simulink model "biadler_sim_3_TEST"  (R2013a)
settings: Solver=ode1  StartTime=0.0  StopTime=5.11  FixedStep=0.001  MaxStep=0.01  RelTol=1e-3
libraries: simulink x4
settings Model: Creator=Administrator  LastModifiedBy=dholley
settings SolverCC: ExtrapolationOrder=1
settings DataIOCC: LimitDataPoints=off  SaveFormat=StructureWithTime  SignalLoggingSaveFormat=ModelDataLogs  SaveOutput=off  SignalLogging=off  DSMLogging=off  SaveTime=off
settings OptimizationCC: InlineParams=on  InlineInvariantSignals=on  ExpressionDepthLimit=2147483647  EfficientFloat2IntCast=on  SimCompilerOptimization=On
settings DebuggingCC: FcnCallInpInsideContextMsg=UseLocalSettings
settings HardwareCC: ProdIntDivRoundTo=Zero  ProdEndianess=LittleEndian  ProdHWDeviceType=Generic->32-bit x86 compatible  TargetIntDivRoundTo=Zero  TargetEndianess=LittleEndian  TargetHWDeviceType=MATLAB Host
settings ModelReferenceCC: ModelReferenceNumInstancesAllowed=Zero
settings RTWCC: SystemTargetFile=grt_malloc.tlc  TemplateMakefile=grt_malloc_default_tmf  Description=Generic Real-Time Target with dynamic memory allocation  RTWVerbose=off  ProcessScript=grt_malloc_make_rtw_hook  RTWCompilerOptimization=On
settings CodeAppCC: GenerateComments=off  SimulinkBlockComments=off
settings GRTTargetCC: CodeReplacementLibrary=C89/C90 (ANSI)  CombineOutputUpdateFcns=off  MatFileLogging=off  GRTInterface=on  UseMalloc=on  ExtModeMexFile=noextcomm

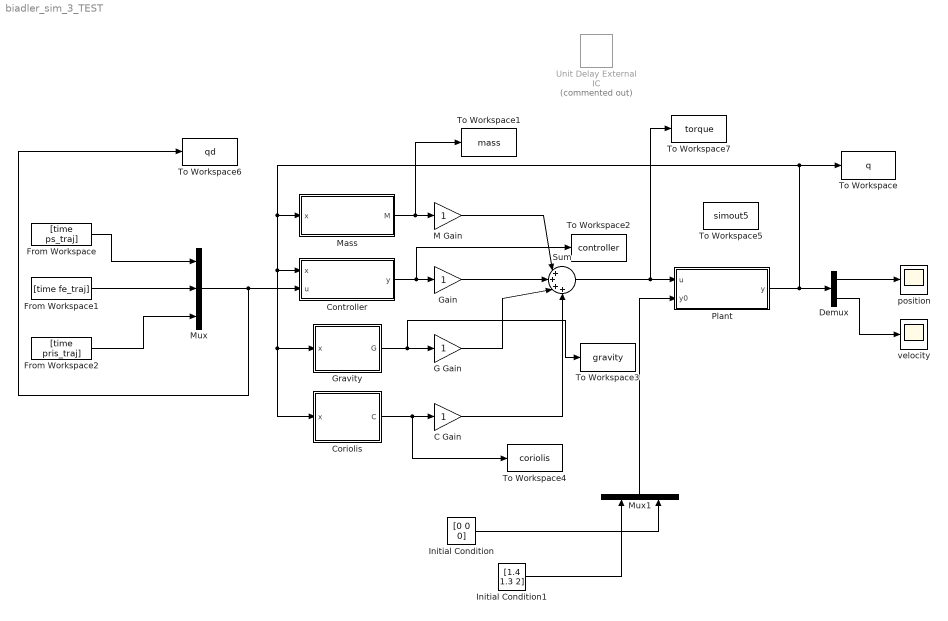
== system biadler_sim_3_TEST ==
  C Gain : Gain
  Controller : Subsystem  TreatAsAtomicUnit=on
  Coriolis : MATLAB Function  TreatAsAtomicUnit=on
  Demux : Demux  Outputs=2
  From Workspace : FromWorkspace  VariableName=[time ps_traj]  SampleTime=0
  From Workspace1 : FromWorkspace  VariableName=[time fe_traj]  SampleTime=0
  From Workspace2 : FromWorkspace  VariableName=[time pris_traj]  SampleTime=0
  G Gain : Gain
  Gain : Gain
  Gravity : MATLAB Function  TreatAsAtomicUnit=on
  Initial Condition : Constant  Value=[0 0 0]
  Initial Condition1 : Constant  Value=[1.4 1.3 2]
  M Gain : Gain
  Mass : Subsystem  TreatAsAtomicUnit=on
  Mux : Mux  Inputs=3
  Mux1 : Mux  Inputs=2
  Plant : Subsystem  TreatAsAtomicUnit=on
  Sum : Sum  Inputs=|++++
  To Workspace : ToWorkspace  VariableName=q  SampleTime=-1  SaveFormat=Timeseries
  To Workspace1 : ToWorkspace  VariableName=mass  SampleTime=-1  SaveFormat=Timeseries
  To Workspace2 : ToWorkspace  VariableName=controller  SampleTime=-1  SaveFormat=Timeseries
  To Workspace3 : ToWorkspace  VariableName=gravity  SampleTime=-1  SaveFormat=Timeseries
  To Workspace4 : ToWorkspace  VariableName=coriolis  SampleTime=-1  SaveFormat=Timeseries
  To Workspace5 : ToWorkspace  VariableName=simout5  SampleTime=-1  SaveFormat=Timeseries
  To Workspace6 : ToWorkspace  VariableName=qd  SampleTime=-1  SaveFormat=Timeseries
  To Workspace7 : ToWorkspace  VariableName=torque  SampleTime=-1  SaveFormat=Timeseries
  Unit Delay External IC : simulink/Additional Math & Discrete/Additional Discrete/Unit Delay External IC  Commented=on  tsamp=-1
  position : Scope
      settings: TickLabels=on  TimeRange=2  YMin=-3  YMax=3  SampleTime=0.05
  velocity : Scope
      settings: TickLabels=on  TimeRange=2  YMin=-1  YMax=1  SampleTime=0.05
  wires:
  Demux/2 -> velocity/1
  Plant/1(y) -> Demux/1, To Workspace/1, Mass/1(x), Controller/1(x), Gravity/1(x), Coriolis/1(x)
  Sum/1 -> To Workspace7/1, Plant/1(u)
  Gravity/1(G) -> To Workspace3/1, G Gain/1
  Coriolis/1(C) -> To Workspace4/1, C Gain/1
  C Gain/1 -> Sum/4
  M Gain/1 -> Sum/1
  G Gain/1 -> Sum/3
  Controller/1(y) -> To Workspace2/1, Gain/1
  Mass/1(M) -> To Workspace1/1, M Gain/1
  Gain/1 -> Sum/2
  Demux/1 -> position/1
  From Workspace/1 -> Mux/1
  From Workspace1/1 -> Mux/2
  From Workspace2/1 -> Mux/3
  Mux/1 -> To Workspace6/1, Controller/2(u)
  Initial Condition/1 -> Mux1/2
  Initial Condition1/1 -> Mux1/1
  Mux1/1 -> Plant/2(y0)

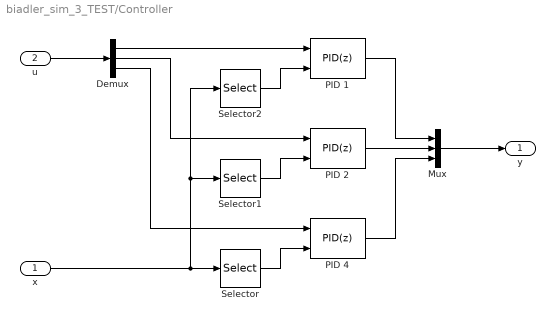
== system biadler_sim_3_TEST/Controller ==
  x : Inport
  u : Inport  Port=2
  Demux : Demux  Outputs=3
  Mux : Mux  Inputs=3
  PID 1 : simulink/Continuous/PID Controller (2DOF)  Controller=PID  TimeDomain=Discrete-time  SampleTime=0.001  IntegratorMethod=Forward Euler  FilterMethod=Forward Euler  Form=Parallel  P=2490  I=3860  D=163  N=250  b=1  c=1  InitialConditionSource=internal  InitialConditionForIntegrator=0  InitialConditionForFilter=0  ExternalReset=none  LimitOutput=off  UpperSaturationLimit=5  LowerSaturationLimit=-5  LinearizeAsGain=off  AntiWindupMode=none  Kb=1  TrackingMode=off  Kt=1  PParamMin=[]  PParamMax=[]  IParamMin=[]  IParamMax=[]  DParamMin=[]  DParamMax=[]  NParamMin=[]  NParamMax=[]  bParamMin=[]  bParamMax=[]  cParamMin=[]  cParamMax=[]  KbParamMin=[]  KbParamMax=[]  KtParamMin=[]  KtParamMax=[]  POutMin=[]  POutMax=[]  IOutMin=[]  IOutMax=[]  DOutMin=[]  DOutMax=[]  NOutMin=[]  NOutMax=[]  bOutMin=[]  bOutMax=[]  cOutMin=[]  cOutMax=[]  KbOutMin=[]  KbOutMax=[]  KtOutMin=[]  KtOutMax=[]  IntegratorOutMin=[]  IntegratorOutMax=[]  FilterOutMin=[]  FilterOutMax=[]  SumOutMin=[]  SumOutMax=[]  Sum1OutMin=[]  Sum1OutMax=[]  Sum2OutMin=[]  Sum2OutMax=[]  Sum3OutMin=[]  Sum3OutMax=[]  SumI1OutMin=[]  SumI1OutMax=[]  SumI2OutMin=[]  SumI2OutMax=[]  SumI3OutMin=[]  SumI3OutMax=[]  SumDOutMin=[]  SumDOutMax=[]  SaturationOutMin=[]  SaturationOutMax=[]  IntegratorContinuousStateAttributes=''  IntegratorStateMustResolveToSignalObject=off  IntegratorRTWStateStorageClass=Auto  FilterContinuousStateAttributes=''  FilterStateMustResolveToSignalObject=off  FilterRTWStateStorageClass=Auto
  PID 2 : simulink/Continuous/PID Controller (2DOF)  Controller=PID  TimeDomain=Discrete-time  SampleTime=0.001  IntegratorMethod=Forward Euler  FilterMethod=Forward Euler  Form=Parallel  P=2490  I=3860  D=163  N=250  b=1  c=1  InitialConditionSource=internal  InitialConditionForIntegrator=0  InitialConditionForFilter=0  ExternalReset=none  LimitOutput=off  UpperSaturationLimit=5  LowerSaturationLimit=-5  LinearizeAsGain=off  AntiWindupMode=none  Kb=1  TrackingMode=off  Kt=1  PParamMin=[]  PParamMax=[]  IParamMin=[]  IParamMax=[]  DParamMin=[]  DParamMax=[]  NParamMin=[]  NParamMax=[]  bParamMin=[]  bParamMax=[]  cParamMin=[]  cParamMax=[]  KbParamMin=[]  KbParamMax=[]  KtParamMin=[]  KtParamMax=[]  POutMin=[]  POutMax=[]  IOutMin=[]  IOutMax=[]  DOutMin=[]  DOutMax=[]  NOutMin=[]  NOutMax=[]  bOutMin=[]  bOutMax=[]  cOutMin=[]  cOutMax=[]  KbOutMin=[]  KbOutMax=[]  KtOutMin=[]  KtOutMax=[]  IntegratorOutMin=[]  IntegratorOutMax=[]  FilterOutMin=[]  FilterOutMax=[]  SumOutMin=[]  SumOutMax=[]  Sum1OutMin=[]  Sum1OutMax=[]  Sum2OutMin=[]  Sum2OutMax=[]  Sum3OutMin=[]  Sum3OutMax=[]  SumI1OutMin=[]  SumI1OutMax=[]  SumI2OutMin=[]  SumI2OutMax=[]  SumI3OutMin=[]  SumI3OutMax=[]  SumDOutMin=[]  SumDOutMax=[]  SaturationOutMin=[]  SaturationOutMax=[]  IntegratorContinuousStateAttributes=''  IntegratorStateMustResolveToSignalObject=off  IntegratorRTWStateStorageClass=Auto  FilterContinuousStateAttributes=''  FilterStateMustResolveToSignalObject=off  FilterRTWStateStorageClass=Auto
  PID 4 : simulink/Continuous/PID Controller (2DOF)  Controller=PID  TimeDomain=Discrete-time  SampleTime=0.001  IntegratorMethod=Forward Euler  FilterMethod=Forward Euler  Form=Parallel  P=2490  I=3860  D=163  N=250  b=1  c=1  InitialConditionSource=internal  InitialConditionForIntegrator=0  InitialConditionForFilter=0  ExternalReset=none  LimitOutput=off  UpperSaturationLimit=5  LowerSaturationLimit=-5  LinearizeAsGain=off  AntiWindupMode=none  Kb=1  TrackingMode=off  Kt=1  PParamMin=[]  PParamMax=[]  IParamMin=[]  IParamMax=[]  DParamMin=[]  DParamMax=[]  NParamMin=[]  NParamMax=[]  bParamMin=[]  bParamMax=[]  cParamMin=[]  cParamMax=[]  KbParamMin=[]  KbParamMax=[]  KtParamMin=[]  KtParamMax=[]  POutMin=[]  POutMax=[]  IOutMin=[]  IOutMax=[]  DOutMin=[]  DOutMax=[]  NOutMin=[]  NOutMax=[]  bOutMin=[]  bOutMax=[]  cOutMin=[]  cOutMax=[]  KbOutMin=[]  KbOutMax=[]  KtOutMin=[]  KtOutMax=[]  IntegratorOutMin=[]  IntegratorOutMax=[]  FilterOutMin=[]  FilterOutMax=[]  SumOutMin=[]  SumOutMax=[]  Sum1OutMin=[]  Sum1OutMax=[]  Sum2OutMin=[]  Sum2OutMax=[]  Sum3OutMin=[]  Sum3OutMax=[]  SumI1OutMin=[]  SumI1OutMax=[]  SumI2OutMin=[]  SumI2OutMax=[]  SumI3OutMin=[]  SumI3OutMax=[]  SumDOutMin=[]  SumDOutMax=[]  SaturationOutMin=[]  SaturationOutMax=[]  IntegratorContinuousStateAttributes=''  IntegratorStateMustResolveToSignalObject=off  IntegratorRTWStateStorageClass=Auto  FilterContinuousStateAttributes=''  FilterStateMustResolveToSignalObject=off  FilterRTWStateStorageClass=Auto
  Selector : Selector  InputPortWidth=6  IndexOptions=Index vector (dialog)  Indices=[3]  OutputSizes=1
  Selector1 : Selector  InputPortWidth=6  IndexOptions=Index vector (dialog)  Indices=[2]  OutputSizes=1
  Selector2 : Selector  InputPortWidth=6  IndexOptions=Index vector (dialog)  Indices=[1]  OutputSizes=1
  y : Outport
  wires:
  Selector2/1 -> PID 1/2
  Selector1/1 -> PID 2/2
  PID 2/1 -> Mux/2
  Mux/1 -> y/1
  PID 1/1 -> Mux/1
  PID 4/1 -> Mux/3
  x/1 -> Selector/1, Selector1/1, Selector2/1
  Demux/3 -> PID 4/1
  Demux/2 -> PID 2/1
  Demux/1 -> PID 1/1
  u/1 -> Demux/1
  Selector/1 -> PID 4/2

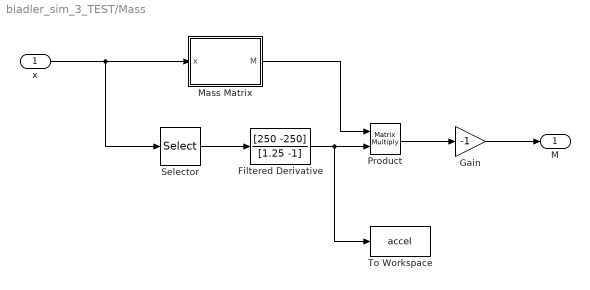
== system biadler_sim_3_TEST/Mass ==
  x : Inport
  Filtered Derivative : DiscreteFilter  Numerator=[250 -250]  Denominator=[1.25 -1]  SampleTime=0.001
  Gain : Gain  Gain=-1
  Mass Matrix : MATLAB Function  TreatAsAtomicUnit=on
  Product : Product  Multiplication=Matrix(*)  RndMeth=Zero
  Selector : Selector  InputPortWidth=6  IndexOptions=Index vector (dialog)  Indices=[4:6]  OutputSizes=1
  To Workspace : ToWorkspace  VariableName=accel  SampleTime=-1  SaveFormat=Timeseries
  M : Outport
  wires:
  x/1 -> Mass Matrix/1(x), Selector/1
  Filtered Derivative/1 -> To Workspace/1, Product/2
  Selector/1 -> Filtered Derivative/1
  Mass Matrix/1(M) -> Product/1
  Product/1 -> Gain/1
  Gain/1 -> M/1

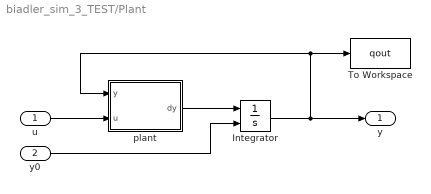
== system biadler_sim_3_TEST/Plant ==
  u : Inport
  y0 : Inport  Port=2
  Integrator : Integrator  InitialConditionSource=external  InitialCondition=[0;0;0.5;0;0;0]
  To Workspace : ToWorkspace  VariableName=qout  SampleTime=-1  SaveFormat=Structure With Time
  plant : MATLAB Function  TreatAsAtomicUnit=on
  y : Outport
  wires:
  Integrator/1 -> y/1, plant/1(y), To Workspace/1
  plant/1(dy) -> Integrator/1
  u/1 -> plant/2(u)
  y0/1 -> Integrator/2

== matlab function biadler_sim_3_TEST/Mass/Mass Matrix ==
  data: x input; M output
function M = fcn(x) %#codegen

I1=[0.38096322, 0.00007420, -0.00044613; 0.00007420, 0.33264110, -0.07673074; -0.00044613, -0.07673074, 0.05442464];
I2=[0.20019857, 0.11214860, -0.00179420; 0.11214860, 0.40696889, -0.00005073; -0.0017942, -0.00005073, 0.57750696];
I3=[0.25101842, -0.00000898, 0.00296055; -0.00000898, 0.24154846, 0.00011129; 0.00296055, 0.00011129, 0.01521556];
I23=I2+I3;

% m2=8.79496939;
m3=3.5;
% rg2=-0.12046546;
% rg3=-0.00429190;
% g=9.80665;

s2=sin(x(2)); c2=cos(x(2));

M=[(I1(3,3)+I23(1,1)*s2^2+I23(2,2)*c2^2-2*I23(1,2)*s2*c2+m3*x(3)*s2), (I23(1,3)*s2-I23(2,3)*c2), 0;
   (I23(1,3)*s2-I23(2,3)*c2), (I23(3,3)+m3*x(3)^2), 0;
   0, 0, m3];

== matlab function biadler_sim_3_TEST/Plant/plant ==
  data: y input; u input; dy output
function dy = fcn(y,u) %#codegen

I1=[0.38096322, 0.00007420, -0.00044613; 0.00007420, 0.33264110, -0.07673074; -0.00044613, -0.07673074, 0.05442464];
I2=[0.20019857, 0.11214860, -0.00179420; 0.11214860, 0.40696889, -0.00005073; -0.0017942, -0.00005073, 0.57750696];
I3=[0.25101842, -0.00000898, 0.00296055; -0.00000898, 0.24154846, 0.00011129; 0.00296055, 0.00011129, 0.01521556];
I23=I2+I3;

m2=8.79496939;
m3=3.5;
rg2=-0.12046546;
rg3=-0.00429190;
g=9.80665;

s2=sin(y(2)); c2=cos(y(2));

dyy=[y(4:6).^2;y(4)*y(5);y(5)*y(6);y(6)*y(4)];
C0=[0, (I23(1,3)*c2+I23(2,3)*s2), 0, (2*(I23(1,1)-I23(2,2))*c2*s2+2*I23(1,2)*(s2^2-c2^2)+m3*y(3)^2*c2), 0, (2*m3*y(3)*s2);
    (-(I23(1,1)-I23(2,2))*c2*s2-I23(1,2)*(s2^2-c2^2)-m3*y(3)^2*c2), 0, 0, 0, (2*m3*y(3)), 0;
    (-m3*y(3)*s2), (-m3*y(3)), 0, 0, 0, 0];
C=C0*dyy;

G=[0;
   -g*(m2*rg2+m3*(rg3+y(3)))*s2;
   m3*g*c2];

M0=[(I1(3,3)+I23(1,1)*s2^2+I23(2,2)*c2^2-2*I23(1,2)*s2*c2+m3*y(3)*s2), (I23(1,3)*s2-I23(2,3)*c2), 0;
   (I23(1,3)*s2-I23(2,3)*c2), (I23(3,3)+m3*y(3)^2), 0;
   0, 0, m3];
M=[eye(3),zeros(3); zeros(3),-M0];

dy=M\[y(4:6);C+G-u];

== matlab function biadler_sim_3_TEST/Coriolis ==
  data: x input; C output
function C = fcn(x) %#codegen

% I1=[0.38096322, 0.00007420, -0.00044613; 0.00007420, 0.33264110, -0.07673074; -0.00044613, -0.07673074, 0.05442464];
I2=[0.20019857, 0.11214860, -0.00179420; 0.11214860, 0.40696889, -0.00005073; -0.0017942, -0.00005073, 0.57750696];
I3=[0.25101842, -0.00000898, 0.00296055; -0.00000898, 0.24154846, 0.00011129; 0.00296055, 0.00011129, 0.01521556];
I23=I2+I3;

% m2=8.79496939;
m3=3.5;
% rg2=-0.12046546;
% rg3=-0.00429190;
% g=9.80665;

s2=sin(x(2)); c2=cos(x(2));

dxx=[x(4:6).^2;x(4)*x(5);x(5)*x(6);x(6)*x(4)];
C0=[0, (I23(1,3)*c2+I23(2,3)*s2), 0, (2*(I23(1,1)-I23(2,2))*c2*s2+2*I23(1,2)*(s2^2-c2^2)+m3*x(3)^2*c2), 0, (2*m3*x(3)*s2);
    (-(I23(1,1)-I23(2,2))*c2*s2-I23(1,2)*(s2^2-c2^2)-m3*x(3)^2*c2), 0, 0, 0, (2*m3*x(3)), 0;
    (-m3*x(3)*s2), (-m3*x(3)), 0, 0, 0, 0];
C=C0*dxx;

== matlab function biadler_sim_3_TEST/Gravity ==
  data: G output; x input
function G = fcn(x) %#codegen

% I1=[0.38096322, 0.00007420, -0.00044613; 0.00007420, 0.33264110, -0.07673074; -0.00044613, -0.07673074, 0.05442464];
% I2=[0.20019857, 0.11214860, -0.00179420; 0.11214860, 0.40696889, -0.00005073; -0.0017942, -0.00005073, 0.57750696];
% I3=[0.25101842, -0.00000898, 0.00296055; -0.00000898, 0.24154846, 0.00011129; 0.00296055, 0.00011129, 0.01521556];
% I23=I2+I3;

m2=8.79496939;
m3=3.5;
rg2=-0.12046546;
rg3=-0.00429190;
g=9.80665;

s2=sin(x(2)); c2=cos(x(2));

G=[0;
   -g*(m2*rg2+m3*(rg3+x(3)))*s2;
   m3*g*c2];
